simulink model "inverted_pendulum_with_interpreted_function"  (R2018a)
settings: Solver=VariableStepAuto  StartTime=0.0  StopTime=30  RelTol=1e-3
values from neighbouring files (symbols this model uses):
  A = [0 1 0 0 ... (first row only)    [lqr_d_cartpend.m]
  A_d = sys_d.A    [lqr_d_cartpend.m]
  B = [0; 1/M; 0; s*1/(M*L)]    [lqr_d_cartpend.m]
  B_d = sys_d.B    [lqr_d_cartpend.m]
  C = [1 1 1 1]    [lqr_d_cartpend.m]
  C_d = sys_d.C    [lqr_d_cartpend.m]
  Ts = 0.1    [lqr_d_cartpend.m]
  y0 = [-3; 0; pi + pi/4; 0]    [lqr_d_cartpend.m]
undefined symbols (not defined in the file or in its folder): Kd, Obd
settings Model: EnablePacing=on  PacingRate=1000  Creator=USER  LastModifiedBy=USER

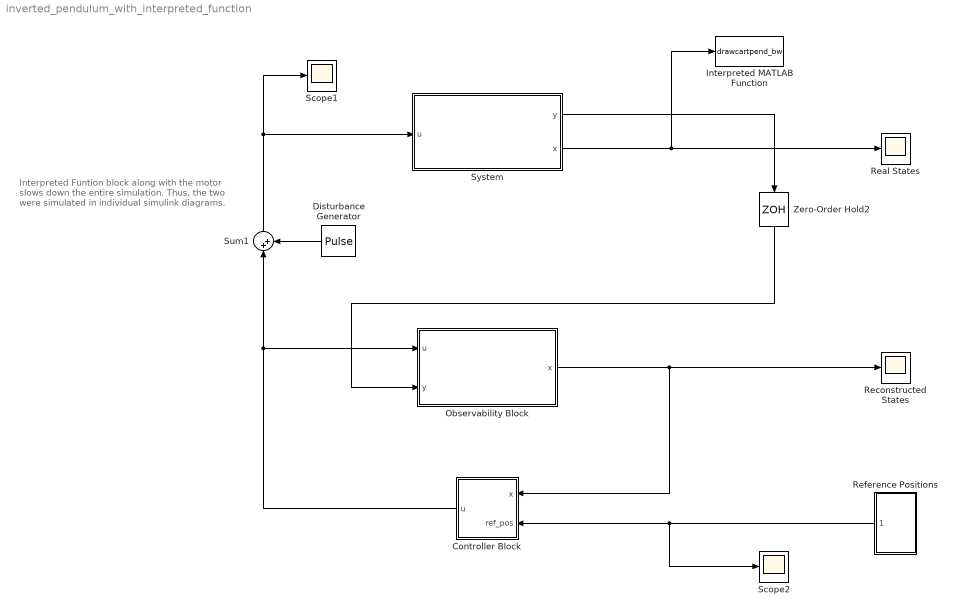
== system inverted_pendulum_with_interpreted_function ==
  note: Interpreted Funtion block along with the motor slows down the entire simulation. Thus, the two were simulated in individual simulink diagrams.
  Controller Block : Subsystem
  Disturbance Generator : DiscretePulseGenerator  PulseType=Time based  Amplitude=10  Period=10  PulseWidth=50
  Interpreted MATLAB Function : MATLABFcn  MATLABFcn=drawcartpend_bw  OutputDimensions=0
  Observability Block : Subsystem
  Real States : Scope
  Reconstructed States : Scope
  Reference Positions : Subsystem
  Scope1 : Scope
  Scope2 : Scope
  Sum1 : Sum  Inputs=|++
  System : Subsystem
  Zero-Order Hold2 : ZeroOrderHold  SampleTime=Ts
  wires:
  Reference Positions/1(ref_pos) -> Controller Block/2(ref_pos), Scope2/1
  Observability Block/1("x ") -> Controller Block/1("x "), Reconstructed States/1
  System/1("y ") -> Zero-Order Hold2/1
  Zero-Order Hold2/1 -> Observability Block/2(y)
  System/2("x ") -> Real States/1, Interpreted MATLAB Function/1
  Controller Block/1("u ") -> Sum1/1, Observability Block/1("u ")
  Disturbance Generator/1 -> Sum1/2
  Sum1/1 -> Scope1/1, System/1("u ")

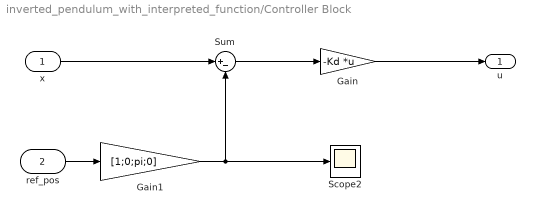
== system inverted_pendulum_with_interpreted_function/Controller Block ==
  "x " : Inport
  ref_pos : Inport  Port=2
  Gain : Gain  Gain=-Kd  Multiplication=Matrix(K*u)
  Gain1 : Gain  Gain=[1;0;pi;0]
  Scope2 : Scope
  Sum : Sum  Inputs=|+-
  "u " : Outport
  wires:
  Gain/1 -> "u "/1
  "x "/1 -> Sum/1
  Sum/1 -> Gain/1
  Gain1/1 -> Scope2/1, Sum/2
  ref_pos/1 -> Gain1/1

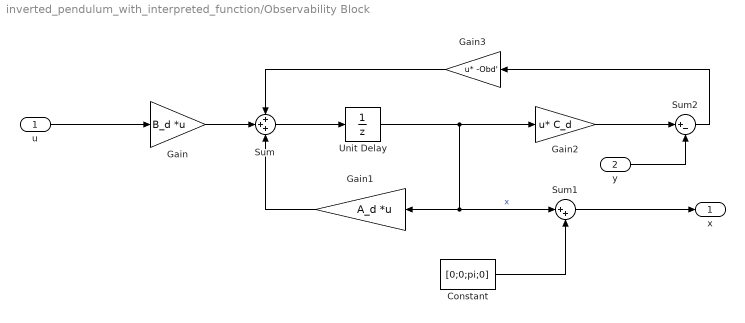
== system inverted_pendulum_with_interpreted_function/Observability Block ==
  "u " : Inport
  y : Inport  Port=2
  Constant : Constant  Value=[0;0;pi;0]
  Gain : Gain  Gain=B_d  Multiplication=Matrix(K*u)
  Gain1 : Gain  Gain=A_d  Multiplication=Matrix(K*u) (u vector)
  Gain2 : Gain  Gain=C_d  Multiplication=Matrix(u*K)
  Gain3 : Gain  Gain=-Obd'  Multiplication=Matrix(u*K)
  Sum : Sum  Inputs=+++
  Sum1 : Sum  Inputs=|++
  Sum2 : Sum  Inputs=|+-
  Unit Delay : UnitDelay  InitialCondition=y0*0  SampleTime=Ts
  "x " : Outport
  wires:
  Sum/1 -> Unit Delay/1
  "u "/1 -> Gain/1
  Gain/1 -> Sum/2
  Unit Delay/1 -> Sum1/1, Gain1/1, Gain2/1  "x"
  Sum1/1 -> "x "/1
  Constant/1 -> Sum1/2
  Gain2/1 -> Sum2/1
  y/1 -> Sum2/2
  Sum2/1 -> Gain3/1
  Gain1/1 -> Sum/3
  Gain3/1 -> Sum/1

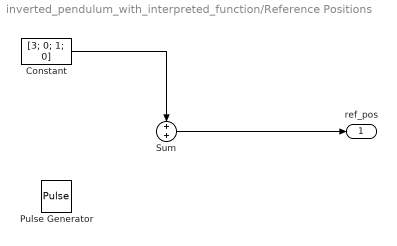
== system inverted_pendulum_with_interpreted_function/Reference Positions ==
  Constant : Constant  Value=[3; 0; 1; 0]
  Pulse Generator : DiscretePulseGenerator  PulseType=Time based  Amplitude=[2;0.3;0;-0.5]  Period=14  PulseWidth=50  PhaseDelay=10
  Sum : Sum
  ref_pos : Outport
  wires:
  Sum/1 -> ref_pos/1
  Constant/1 -> Sum/1

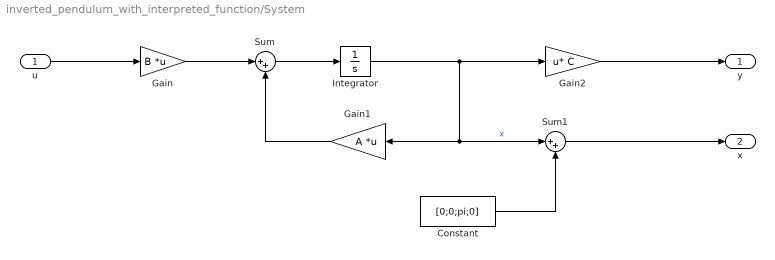
== system inverted_pendulum_with_interpreted_function/System ==
  "u " : Inport
  Constant : Constant  Value=[0;0;pi;0]
  Gain : Gain  Gain=B  Multiplication=Matrix(K*u)
  Gain1 : Gain  Gain=A  Multiplication=Matrix(K*u) (u vector)
  Gain2 : Gain  Gain=C  Multiplication=Matrix(u*K)
  Integrator : Integrator  InitialCondition=[-3; -0.3; pi/10*4; 0.5]
  Sum : Sum  Inputs=|++
  Sum1 : Sum  Inputs=|++
  "y " : Outport
  "x " : Outport  Port=2
  wires:
  Sum/1 -> Integrator/1
  "u "/1 -> Gain/1
  Gain/1 -> Sum/1
  Gain1/1 -> Sum/2
  Gain2/1 -> "y "/1
  Integrator/1 -> Gain2/1, Sum1/1, Gain1/1  "x"
  Sum1/1 -> "x "/1
  Constant/1 -> Sum1/2
